simulink model "Khajuriwala_Rishi_RBE_501_HW_04_question2_b_sim"  (R2017b)
settings: Solver=VariableStepAuto  StartTime=0.0  StopTime=10.0  RelTol=1e-3
values from neighbouring files (symbols this model uses):
  a1 = 150    [Khajuriwala_Rishi_RBE501_HW2_Inverse_kinematics.m]    (also in Khajuriwala_Rishi_RBE501_HW2_Jacobian.m = sym('a1','real'); Khajuriwala_rishi_RBE_501_Hw2_Workspace.m = 0; Khajuriwala_rishi_rbe_501_HW_03_question_2_matlab.m = sym('a1','real'))
  a2 = 600    [Khajuriwala_Rishi_RBE501_HW2_Inverse_kinematics.m]    (also in Khajuriwala_Rishi_RBE501_HW2_Jacobian.m = sym('a2','real'); Khajuriwala_rishi_RBE_501_Hw2_Workspace.m = 150; Khajuriwala_rishi_rbe_501_HW_03_question_2_matlab.m = sym('a2','real'))
settings Model: Creator=rishi  LastModifiedBy=rishi

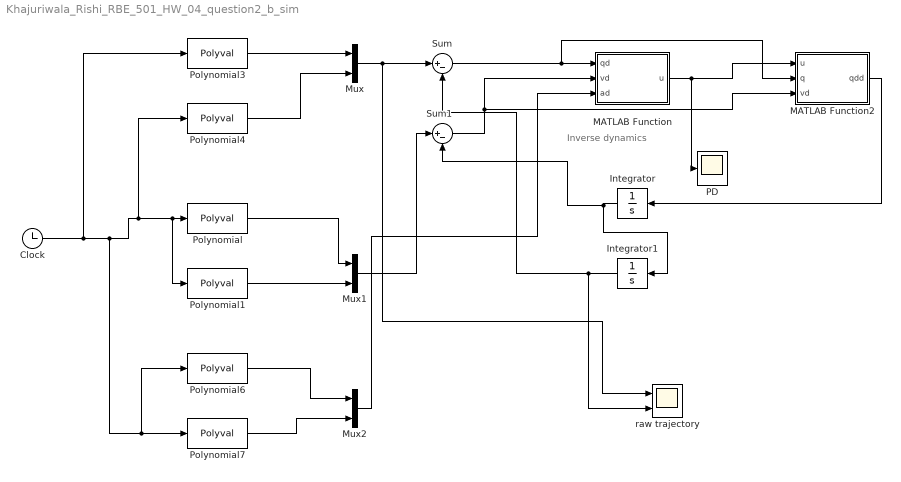
== system Khajuriwala_Rishi_RBE_501_HW_04_question2_b_sim ==
  note: Inverse dynamics
  Clock : Clock
  Integrator : Integrator
  Integrator1 : Integrator
  MATLAB Function : MATLAB Function  TreatAsAtomicUnit=on
  MATLAB Function2 : MATLAB Function  TreatAsAtomicUnit=on
  Mux : Mux  Inputs=2
  Mux1 : Mux  Inputs=2
  Mux2 : Mux  Inputs=2
  "PD " : Scope
  Polynomial : Polyval  Coefs=[a1(2) 2*a1(3) 3*a1(4)]
  Polynomial1 : Polyval  Coefs=[a2(2) 2*a2(3) 3*a2(4)]
  Polynomial3 : Polyval  Coefs=[ a1(1) a1(2) a1(3) a1(4)]
  Polynomial4 : Polyval  Coefs=[ a2(1) a2(2) a2(3) a2(4)]
  Polynomial6 : Polyval  Coefs=[2*a1(3) 6*a1(4)]
  Polynomial7 : Polyval  Coefs=[2*a2(3) 6*a2(4)]
  Sum : Sum  Inputs=|+-
  Sum1 : Sum  Inputs=|+-
  "raw trajectory " : Scope  NumInputPorts=2
  wires:
  Mux/1 -> Sum/1, "raw trajectory "/1
  Polynomial4/1 -> Mux/2
  Integrator/1 -> Sum1/2, Integrator1/1
  Mux1/1 -> Sum1/1
  Polynomial6/1 -> Mux2/1
  Polynomial7/1 -> Mux2/2
  Sum1/1 -> MATLAB Function2/3(vd), MATLAB Function/2(vd)
  Clock/1 -> Polynomial3/1, Polynomial7/1, Polynomial6/1, Polynomial4/1, Polynomial1/1, Polynomial/1
  Polynomial/1 -> Mux1/1
  Integrator1/1 -> "raw trajectory "/2, Sum/2
  Polynomial3/1 -> Mux/1
  Mux2/1 -> MATLAB Function/3(ad)
  Sum/1 -> MATLAB Function2/2(q), MATLAB Function/1(qd)
  MATLAB Function2/1(qdd) -> Integrator/1
  Polynomial1/1 -> Mux1/2
  MATLAB Function/1(u) -> "PD "/1, MATLAB Function2/1(u)

== matlab function Khajuriwala_Rishi_RBE_501_HW_04_question2_b_sim/MATLAB Function ==
  data: qd input; u output; vd input; ad input
function u = fcn(qd, vd, ad)

INVERSE DYNAMICS CONTROLLER
function u = fcn(qd, vd, ad)
Kv = diag([1 1 1]); 
Kp = diag([1 1 1]);
ad = transpose(ad);

aq = transpose(ad - transpose(Kv*(vd)) - transpose(Kp*(qd)))
 [M,C,G]=dynamics();

u = M*aq + C*vd + G;
function[M,C,G]= dynamics()
syms theta1 theta2  L1 L2 
DH =[[0,  pi/2, L1, theta1]
     [L2, 0,    0,  theta2] ;

theta = [theta1,theta2];
d = [L1,0];
alpha =[pi/2,0];
a = [0,L2];
 %% Frame transformations
T1 = Fk(t(1),d(1),alpha(1),a(1));
T2 = Fk(t(2),d(2),alpha(2),a(2));
  
 
 
 T01 = T1;
 T02 = simplify(T01*T2);
  
J1= simplify(jacobian(T01(1:3,4),[theta1]));
J2= simplify(jacobian(T02(1:3,4),[theta1 theta2]));


syms dq1 dq2  
v_m1 = simplify(J1 * dq1);
v_m2 = simplify(J2 * [dq1;dq2]);


syms m1 m2 
k1 =simplify(( 0.5 * m1 * (v_m1.' * v_m1)));
k2 =simplify(( 0.5 * m2 * (v_m2.' * v_m2)));


K = k1 +k2 ;

g = 9.8;

P1 = simplify(m1 * g * T01(3,4));
P2 = simplify(m2 * g * T02(3,4));


P = P1 + P2  ;

L = simplify ( K - P );
syms th1(t) th2(t) 
syms ddq1 ddq2 

dL_dq1 = diff(L,dq1);
dL_dq1_sub= subs(dL_dq1,[theta1 theta2 dq1 dq2],[th1 th2 diff(th1(t),t) diff(th2(t),t)]);
dL1 = diff(dL_dq1_sub,t);
dL1_a = subs(dL1,[th1 th2 diff(th1(t),t) diff(th2(t),t) diff(th1(t),t,t) diff(th2(t),t,t)],[theta1 theta2 dq1 dq2 ddq1 ddq2]);
dL_dq2 = diff(L,dq2);
dL_dq2_sub= subs(dL_dq2,[theta1 theta2 dq1 dq2],[th1 th2 diff(th1(t),t) diff(th2(t),t)]);
dL2 = diff(dL_dq2_sub,t);
dL2_a = subs(dL2,[th1 th2 diff(th1(t),t) diff(th2(t),t) diff(th1(t),t,t) diff(th2(t),t,t)],[theta1 theta2 dq1 dq2 ddq1 ddq2]);
     
dL1_b = diff(L,theta1);
dL2_b = diff(L,theta2);


Tau1 = dL1_a - dL1_b;
Tau2 = dL2_a - dL2_b;

%% m matrix
M11 = simplify(Tau1 - subs(Tau1,ddq1,0))/ddq1;
M12 = simplify(Tau1 - subs(Tau1,ddq2,0))/ddq2;

M21 = simplify(Tau2 - subs(Tau2,ddq1,0))/ddq1;
M22 = simplify(Tau2 - subs(Tau2,ddq2,0))/ddq2;


M = simplify([M11 M12 ;
              M21 M22]) ;
%% G matrix    
G1 = subs(Tau1, [dq1 dq2 ddq1 ddq2],[0 0 0 0]);
G2 = subs(Tau2, [dq1 dq2 ddq1 ddq2],[0 0 0 0]);


G = simplify([G1;G2]);
%% C matrix
C1 = Tau1- (M(1,:)* [ddq1 ddq2 ddq3].' + G1);
C2 = Tau2- (M(2,:)* [ddq1 ddq2 ddq3].' + G2);


C = simplify([C1;C2]);


function [ transMatrix ] =Fk(t,d,alpha,a)
    rotOldZAxis = [cos(t) -sin(t) 0 0;...
    sin(t) cos(t) 0 0;...
    0 0 1 0;...
    0 0 0 1];
    translationOldZAxis = [1 0 0 0;...
    0 1 0 0;...
    0 0 1 d;...
    0 0 0 1];
    translationNewXAxis = [1 0 0 a;...
    0 1 0 0;...
    0 0 1 0;...
    0 0 0 1];
    rotNewXAxis = [1 0 0 0;...
    0 cos(alpha) -sin(alpha) 0;...
    0 sin(alpha) cos(alpha) 0;...
    0 0 0 1];

    transMatrix = rotOldZAxis*translationOldZAxis*translationNewXAxis*rotNewXAxis;
end
end
end

== matlab function Khajuriwala_Rishi_RBE_501_HW_04_question2_b_sim/MATLAB Function2 ==
  data: u input; qdd output; q input; vd input
function qdd = dynamics(u, q, vd)
DYNAMICS FUNCTION
function qdd   = dynamics(u,q,vd)



syms theta1 theta2  L1 L2 
DH =[[0,  pi/2, L1, theta1]
     [L2, 0,    0,  theta2] 
 %% Frame transformations
 T1 = FrameTransform(DH(1,:));
 T2 = FrameTransform(DH(2,:));
 
 
 T01 = T1;
 T02 = simplify(T01*T2);
  
J1= simplify(jacobian(T01(1:3,4),[theta1]));
J2= simplify(jacobian(T02(1:3,4),[theta1 theta2]));


syms dq1 dq2  
v_m1 = simplify(J1 * dq1);
v_m2 = simplify(J2 * [dq1;dq2]);


syms m1 m2 
k1 =simplify(( 0.5 * m1 * (v_m1.' * v_m1)));
k2 =simplify(( 0.5 * m2 * (v_m2.' * v_m2)));


K = k1 +k2 ;

g = 9.8;

P1 = simplify(m1 * g * T01(3,4));
P2 = simplify(m2 * g * T02(3,4));


P = P1 + P2  ;

L = simplify ( K - P );
syms th1(t) th2(t) 
syms ddq1 ddq2 

dL_dq1 = diff(L,dq1);
dL_dq1_sub= subs(dL_dq1,[theta1 theta2 dq1 dq2],[th1 th2 diff(th1(t),t) diff(th2(t),t)]);
dL1 = diff(dL_dq1_sub,t);
dL1_a = subs(dL1,[th1 th2 diff(th1(t),t) diff(th2(t),t) diff(th1(t),t,t) diff(th2(t),t,t)],[theta1 theta2 dq1 dq2 ddq1 ddq2]);
dL_dq2 = diff(L,dq2);
dL_dq2_sub= subs(dL_dq2,[theta1 theta2 dq1 dq2],[th1 th2 diff(th1(t),t) diff(th2(t),t)]);
dL2 = diff(dL_dq2_sub,t);
dL2_a = subs(dL2,[th1 th2 diff(th1(t),t) diff(th2(t),t) diff(th1(t),t,t) diff(th2(t),t,t)],[theta1 theta2 dq1 dq2 ddq1 ddq2]);
     
dL1_b = diff(L,theta1);
dL2_b = diff(L,theta2);


Tau1 = dL1_a - dL1_b;
Tau2 = dL2_a - dL2_b;

%% m matrix
M11 = simplify(Tau1 - subs(Tau1,ddq1,0))/ddq1;
M12 = simplify(Tau1 - subs(Tau1,ddq2,0))/ddq2;

M21 = simplify(Tau2 - subs(Tau2,ddq1,0))/ddq1;
M22 = simplify(Tau2 - subs(Tau2,ddq2,0))/ddq2;


M = simplify([M11 M12 ;
              M21 M22]) ;
%% G matrix    
G1 = subs(Tau1, [dq1 dq2 ddq1 ddq2],[0 0 0 0]);
G2 = subs(Tau2, [dq1 dq2 ddq1 ddq2],[0 0 0 0]);


G = simplify([G1;G2]);
%% C matrix
C1 = Tau1- (M(1,:)* [ddq1 ddq2 ddq3].' + G1);
C2 = Tau2- (M(2,:)* [ddq1 ddq2 ddq3].' + G2);


C = simplify([C1;C2]);


function [ x ] = FrameTransform( y )
a = y(1);
alpha = y(2) * (pi/180);
d = y(3);
theta = y(4) * (pi/180);
RotzTheta = [cos(theta), -sin(theta), 0, 0;
             sin(theta), cos(theta), 0, 0;
            0, 0, 1, 0;
            0, 0, 0, 1];
TranszD = [1, 0, 0, 0;
            0, 1, 0, 0;
            0, 0, 1, d;
            0, 0, 0, 1];
TransxA = [1,0,0,a;
           0,1,0,0;
           0,0,1,0;
           0,0,0,1];
RotxAlpha = [1,0,0,0;
             0, cos(alpha), -sin(alpha), 0;
             0 sin(alpha), cos(alpha), 0;
             0,0, 0, 1];
x = RotzTheta * TranszD * TransxA * RotxAlpha;


qdd =  inv(M)*(u - C*vd - G);
end    
end
